simulink subsystem "PowerModuleLoss"  (R2023b)
settings: Solver=VariableStepAuto  StartTime=0.0  StopTime=10.0  RelTol=1e-3
values from neighbouring files (symbols this model uses):
  inverter = {}    [init_file.m]
  motor = {}    [init_file.m]
settings Model: Creator=benli  LastModifiedBy=benli

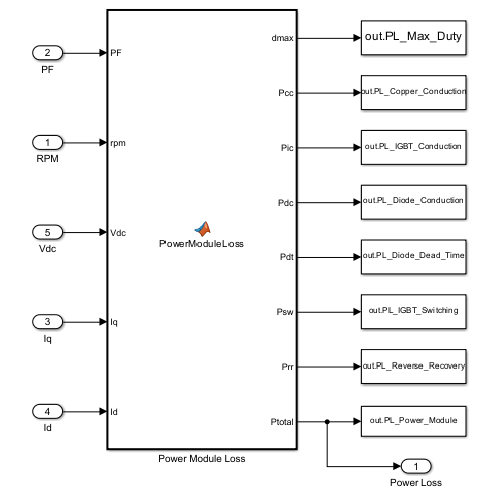
[thumbnail: Simulink's stored preview of the top-level diagram]
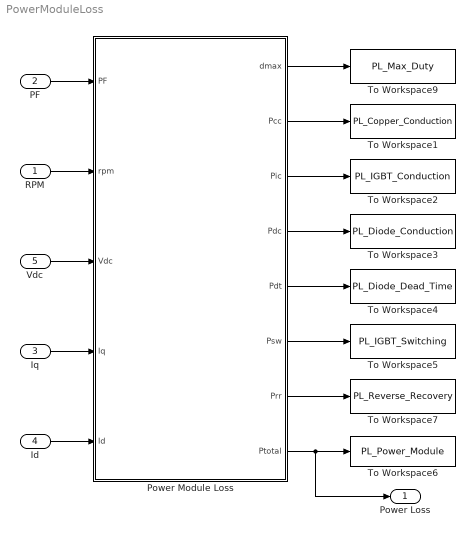
== system PowerModuleLoss ==
  RPM : Inport
  PF : Inport  Port=2
  Iq : Inport  Port=3  OutDataTypeStr=double
  Id : Inport  Port=4  OutDataTypeStr=double
  Vdc : Inport  Port=5
  Power Module Loss : MATLAB Function  TreatAsAtomicUnit=on
  To Workspace1 : ToWorkspace  VariableName=PL_Copper_Conduction  SampleTime=-1
  To Workspace2 : ToWorkspace  VariableName=PL_IGBT_Conduction  SampleTime=-1
  To Workspace3 : ToWorkspace  VariableName=PL_Diode_Conduction  SampleTime=-1
  To Workspace4 : ToWorkspace  VariableName=PL_Diode_Dead_Time  SampleTime=-1
  To Workspace5 : ToWorkspace  VariableName=PL_IGBT_Switching  SampleTime=-1
  To Workspace6 : ToWorkspace  VariableName=PL_Power_Module  SampleTime=-1
  To Workspace7 : ToWorkspace  VariableName=PL_Reverse_Recovery  SampleTime=-1
  To Workspace9 : ToWorkspace  VariableName=PL_Max_Duty  SampleTime=-1
  Power Loss : Outport
  wires:
  Iq/1 -> Power Module Loss/4(Iq)
  Id/1 -> Power Module Loss/5(Id)
  RPM/1 -> Power Module Loss/2(rpm)
  PF/1 -> Power Module Loss/1(PF)
  Vdc/1 -> Power Module Loss/3(Vdc)
  Power Module Loss/8(Ptotal) -> Power Loss/1, To Workspace6/1
  Power Module Loss/2(Pcc) -> To Workspace1/1
  Power Module Loss/3(Pic) -> To Workspace2/1
  Power Module Loss/4(Pdc) -> To Workspace3/1
  Power Module Loss/5(Pdt) -> To Workspace4/1
  Power Module Loss/6(Psw) -> To Workspace5/1
  Power Module Loss/7(Prr) -> To Workspace7/1
  Power Module Loss/1(dmax) -> To Workspace9/1

== matlab function PowerModuleLoss/Power Module Loss ==
  data: dmax output; Pcc output; PF input; rpm input; Pic output; Vdc input; Pdc output; Pdt output; Psw output; Prr output; Iq input; Id input; inverter parameter; motor parameter; Ptotal output
function [dmax, Pcc, Pic, Pdc, Pdt, Psw, Prr, Ptotal] = PowerModuleLoss(PF, rpm, Vdc, Iq, Id, inverter, motor)

    %% Struct parameters

    % Inverter parameters

    fsw = inverter.fsw;                             % AMK inverter switching frequency
    n_igbt = inverter.n_igbt;                       % IGBT switching loss sensitivity
    sw_i = inverter.swi_x_swe_y(:,1);               % Switching current LUT index
    sw_e = inverter.swi_x_swe_y(:,2);               % Switching energy LUT value
    rr_i = inverter.rri_x_rre_y(:,1);               % Reverse recovery current LUT index
    rr_e = inverter.rri_x_rre_y(:,2);               % Reverse recovery energy LUT value
    c_i = inverter.ci_x_cp_y(:,1);                  % IGBT conduction current LUT index
    c_p = inverter.ci_x_cp_y(:,2);                  % IGBT conduction power LUT value
    d_i = inverter.di_x_dp_y(:,1);                  % Diode current LUT index
    d_p = inverter.di_x_dp_y(:,2);                  % Diode power LUT value
    td = inverter.dt_duty;                          % Dead time duty
    Vref = inverter.Vref;                           % Switching loss reference voltage
    Rccee = inverter.Rccee;                         % Collector + emitter resistance
    n = inverter.n_sample;                          % Number of loss samples

    % Motor parameters

    Ld = motor.Ld;                                  % D-axis inductance
    Lq = motor.Lq;                                  % Q-axis inductance
    Lambda_m = motor.Lambda_m;                      % Flux linkage
    Rw = motor.Rw;                                  % Winding resistance
    Pp = motor.Pp;                                  % Pole pairs
    
    %% Rotational parameters

    we = (rpm * Pp * pi)/30;                        % Electric angular frequency
    a = linspace(0, pi, n+1);                       % Sample angle array
    phi = acosd(PF);                                % Phase delay
    
    %% DQ0 frame

    Vd = Rw * Id - we * Lq * Iq;                    % D-axis voltage
    Vq = Rw * Iq + we * (Ld * Id + Lambda_m);       % Q-axis voltage

    %% ABC frame

    % SPWM

    SPWM_Va = Vq*cos(a) + Vd*sin(a);                % Phase a sinusoidal voltage
    SPWM_Vb = Vq*cos(a+2*pi/3) + Vd*sin(a+2*pi/3);  % Phase b sinusoidal voltage
    SPWM_Vc = Vq*cos(a+4*pi/3) + Vd*sin(a+4*pi/3);  % Phase c sinusoidal voltage

    % SVM

    % Zero sequence voltage
    Vz = -(min([SPWM_Va; SPWM_Vb; SPWM_Vc])+max([SPWM_Va; SPWM_Vb; SPWM_Vc]))/2;

    Va = abs(SPWM_Va + Vz);                         % Phase a voltage sample
    Ia = abs(Iq*cos(a-phi) + Id*sin(a-phi));        % Phase a current sample

    %% Switching Parameters
    
    d = Va/Vdc + 0.5;                               % Half bridge duty cycle
    dmax = max(d);                                  % Max duty cycle
    d(d>1) = 1;                                     % Restrict duty cycle to 1

    Cv = Vdc/Vref;                                  % Voltage loss scaling constant

    ta = 1-td;                                      % Half bridge alive time

    %% Power Module Loss
    
    % Intermediate diode power loss array
    Pd = interp1(d_i, d_p, Ia(1:n));

    % 3 phase half-bridge losses

    % Copper conduction loss
    Pcc = 1.5 * Rccee * (Id^2 + Iq^2);

    % IGBT conduction loss
    Pic = 3/n * ta * interp1(c_i, c_p, Ia(1:n)) * d(1:n)';

    % FWD conduction loss
    Pdc = 3/n * ta * Pd * (1 - d(1:n))';

    % FWD dead time loss
    Pdt = 3/n * td * sum(Pd);

    % Switching losses
    Psw = 3/n * fsw * sum(interp1(sw_i, sw_e, Ia(1:n)) * Cv^n_igbt);

    % Reverse recovery losses
    Prr = 3/n * fsw * sum(interp1(rr_i, rr_e, Ia(1:n)) * Cv^0.6);

    % Total inverter losses
    Ptotal = Pcc + Pic + Pdc + Pdt + Psw + Prr;
    
end
